simulink model "Sim_Multi"  (R2019b)
settings: Solver=VariableStepAuto  StartTime=0.0  StopTime=sim_time  FixedStep=t_sim  MaxStep=t_control  RelTol=1e-5  EnableMultiTasking=on
model workspace (MAT data in the model file):
  start_time = 1
values from neighbouring files (symbols this model uses):
  Att_init = [0;0;0] * d2r    [Init_Multi.m]
  Blade_flapping = 0    [Init_Multi.m]
  C_D = 0.40    (= 0.4)    [Init_Multi.m]
  CoG_nominal = [0;0;0.001]    [Init_Multi.m]
  CoG_real = [0;0;0.001]    [Init_Multi.m]
  Coriolis_correction = 0    [Init_Multi.m]
  d2r = pi/180    (= 0.0174532925199)    [Init_Multi.m]
  Dyn_thrust = 0    [Init_Multi.m]
  g = 9.80665    [Init_Multi.m]
  J_nominal = [Jxx Jxy Jxz;Jyx Jyy Jyz;Jzx Jzy Jzz]    [Init_Multi.m]
  J_real = [Jxx Jxy Jxz;Jyx Jyy Jyz;Jzx Jzy Jzz]    [Init_Multi.m]
  k1 = -1.125    [Init_Multi.m]
  k2 = -1.372    [Init_Multi.m]
  k3 = -1.718    [Init_Multi.m]
  k4 = -0.655    [Init_Multi.m]
  k_a1s = 1.5 / 4.0    (= 0.375)    [Init_Multi.m]
  k_beta = 0.23    [Init_Multi.m]
  kappa = 1.00    (= 1)    [Init_Multi.m]
  mass_nominal = 0.550    (= 0.55)    [Init_Multi.m]
  mass_real = 0.550    (= 0.55)    [Init_Multi.m]
  max_thrust = max_thrust + (MotorMatrix_nominal(i,7)*MotorMatrix_nominal(i,12)+MotorMatrix_nominal(i,8)*MotorMatrix_nominal(i,12)^2)    [Init_Multi.m]
  MaxRate_cmd = [360;360;120] * d2r    [Init_Multi.m]
  min_thrust = min_thrust + (MotorMatrix_nominal(i,7)*MotorMatrix_nominal(i,11)+MotorMatrix_nominal(i,8)*MotorMatrix_nominal(i,11)^2)    [Init_Multi.m]
  MotorMap = B' * inv(B * B')    [Init_Multi.m]
  MotorMatrix_nominal = [045 , 0.170 , -0.028 , -1 , 1.0 , 0.010 , [9.6820 , 0.010872]*1e-5 , [1.4504 , 0.0016312]*1e-6 , 0000 , 6000 , [0.0 , 0.0 , 0.0] , 8*2.54/100 , 11/1000;                         135 , 0.170 , -0.028 , +1 , 1.0 , 0.010 , [9.6820 , 0.010872]*1e-5 , [1.4504 , 0.0016312]*1e-6 , 0000 , 6000 , [0.0 , 0.0 , 0.0] , 8*2.54/100 , 11/1000;                         225 , 0.170 , -0.028 , -1 , 1.0 , 0.010 , [9. ...(+284 chars)    [Init_Multi.m]
  MotorMatrix_real = [045 , 0.170 , -0.028 , -1 , 1.0 , 0.010 , [9.6820 , 0.010872]*1e-5 , [1.4504 , 0.0016312]*1e-6 , 0000 , 6000 , [0.0 , 0.0 , 0.0] , 8*2.54/100 , 11/1000;                      135 , 0.170 , -0.028 , +1 , 1.0 , 0.010 , [9.6820 , 0.010872]*1e-5 , [1.4504 , 0.0016312]*1e-6 , 0000 , 6000 , [0.0 , 0.0 , 0.0] , 8*2.54/100 , 11/1000;                      225 , 0.170 , -0.028 , -1 , 1.0 , 0.010 , [9.6820 , ...(+275 chars)    [Init_Multi.m]
  Noise_flag = 1    [Init_Multi.m]
  omega_init = [0;0;0]    [Init_Multi.m]
  q_init = rpy2quat(Att_init)    [Init_Multi.m]
  r2d = 180/pi    (= 57.2957795131)    [Init_Multi.m]
  rho = 1.225    [Init_Multi.m]
  rpm2radpersec = 2*pi/60    (= 0.10471975512)    [Init_Multi.m]
  rpm_init = 3104.5025852    [Init_Multi.m]
  Surface_params = [a;b;c]    [Init_Multi.m]
  t_control = t_control_2*4    (= 0.02)    [Init_Multi.m]
  t_sim = 1/1000    (= 0.001)    [Init_Multi.m]
  thrust_reserve = 0.10    (= 0.1)    [Init_Multi.m]
  v_h = 4.0    (= 4)    [Init_Multi.m]
  Vb_init = [0;0;0]    [Init_Multi.m]
  Vi_init = R_IB_init' * Vb_init    [Init_Multi.m]
  Xi_init = [0;0;-1]    [Init_Multi.m]
undefined symbols (not defined in the file or in its folder): anti_windup_1, anti_windup_2, DiscIntNeverNeededParam, Kd_1, Kd_2, Kff_1, Kff_2, Ki_1, Ki_2, Kp_1, Kp_2, Kpass_1, magnitude, rpy2quat, thrust2rpm
libraries: simulink x35, dspsigops x3, sharedtransform x2, dspmtrx3 x1, robotuavlib x1, vrlib x1
(part 1 of 4)
settings Model: SimulationMode=accelerator  Creator=JV  LastModifiedBy=max_g
settings DataIOCC: LimitDataPoints=on  SaveFormat=Array  ReturnWorkspaceOutputs=off
settings OptimizationCC: ExpressionDepthLimit=2147483647  InitFltsAndDblsToZero=on  LifeSpan=inf
settings DebuggingCC: UnderspecifiedInitializationDetection=Classic  MergeDetectMultiDrivingBlocksExec=none  SolverPrmCheckMsg=warning  FcnCallInpInsideContextMsg=warning  StateNameClashWarn=warning  SFUnexpectedBacktrackingDiag=warning  SFNoUnconditionalDefaultTransitionDiag=warning  SFExecutionAtInitializationDiag=none  ArithmeticOperatorsInVariantConditions=warning
settings HardwareCC: ProdBitPerPointer=32  ProdBitPerSizeT=32  ProdBitPerPtrDiffT=32  ProdLargestAtomicFloat=None  ProdIntDivRoundTo=Undefined  ProdEndianess=Unspecified  ProdWordSize=32  ProdHWDeviceType=32-bit Generic
settings ModelReferenceCC: PropagateSignalLabelsOutOfModel=off
settings SFSimCC: SimUseLocalCustomCode=off  CustomCodeUndefinedFunction=UseInterfaceOnly
settings RTWCC: RTWUseLocalCustomCode=off
settings CodeAppCC: StateflowObjectComments=on
settings GRTTargetCC: TargetLangStandard=C89/C90 (ANSI)  GeneratePreprocessorConditionals=Disable all  CombineOutputUpdateFcns=off  GRTInterface=on
settings ConfigComp: CovMetricSettings=dw  CovHtmlReporting=on  CovSaveCumulativeToWorkspaceVar=on  CovSaveSingleToWorkspaceVar=on  CovExternalEMLEnable=off  CovSFcnEnable=off

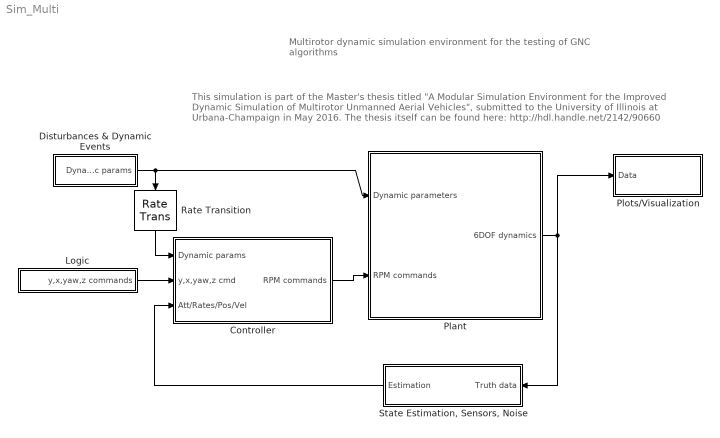
== system Sim_Multi ==
  note: This simulation is part of the Master's thesis titled "A Modular Simulation Environment for the Improved Dynamic Simulation
      | of Multirotor Unmanned Aerial Vehicles", submitted to the University of Illinois at Urbana-Champaign in May 2016.
      | The thesis itself can be found here: http://hdl.handle.net/2142/90660
  note: Multirotor dynamic simulation environment
      | for the testing of GNC algorithms
  Controller : Subsystem
  Disturbances & Dynamic Events : Subsystem
  Logic : Subsystem
  Plant : Subsystem
  Plots/Visualization : Subsystem
  Rate Transition : RateTransition  OutPortSampleTime=t_control_2
  "State Estimation, Sensors, Noise" : Subsystem
  wires:
  Plant/1(6DOF dynamics) -> "State Estimation, Sensors, Noise"/1(Truth data), Plots/Visualization/1(Data)
  Logic/1(y,x,yaw,z commands) -> Controller/2(y,x,yaw,z cmd)
  "State Estimation, Sensors, Noise"/1(Estimation) -> Controller/3(Att/Rates/Pos/Vel)
  Controller/1(RPM commands) -> Plant/2(RPM commands)
  Disturbances & Dynamic Events/1(Dynamic params) -> Plant/1(Dynamic parameters), Rate Transition/1
  Rate Transition/1 -> Controller/1(Dynamic params)

== system Sim_Multi/Controller ==
  note: All system parameters used in this block are the nominal parameters
      | that the controller is given about the system.
      | The true parameters of the dynamic system such as mass, inertia,
      | motor mapping matrix, ... may differ from these values.
  Dynamic params : Inport
  y,x,yaw,z cmd : Inport  Port=2
  Att/Rates/Pos/Vel : Inport  Port=3
  Controller Structure : Subsystem
  Mapping thrust to rpm and saturation : Subsystem
  Motor mapping : Subsystem
  Reshape : Reshape  OutputDimensionality=Column vector (2-D)
  RPM commands : Outport
  tag scope: RPM_commands=global
  wires:
  Att/Rates/Pos/Vel/1 -> Controller Structure/2(Att/Rates/Pos/Vel)
  Controller Structure/1(Torques/thrust cmd) -> Motor mapping/1(Torques/thrust cmd)
  y,x,yaw,z cmd/1 -> Controller Structure/1(y,x,yaw,z cmd)
  Reshape/1 -> RPM commands/1
  Dynamic params/1 -> Controller Structure/3(Dynamic params), Mapping thrust to rpm and saturation/2(Dynamic parameters)
  Mapping thrust to rpm and saturation/1(RPM_cmd) -> [RPM_commands], Reshape/1
  Motor mapping/1(Thrust cmds) -> Mapping thrust to rpm and saturation/1(Thrust_cmds)

== system Sim_Multi/Disturbances & Dynamic Events ==
  Bus Creator : BusCreator  Inputs=12
  Constant : Constant  Value=MotorMatrix_real
  Constant1 : Constant  Value=CoG_real
  Constant2 : Constant  Value=mass_real
  Constant3 : Constant  Value=J_real
  Constant4 : Constant  Value=MotorMatrix_nominal
  Constant5 : Constant  Value=CoG_nominal
  Constant6 : Constant  Value=mass_nominal
  Constant7 : Constant  Value=J_nominal
  Disturbance (forces) : Constant  Value=0*[1;1;1]
  Disturbance (torques) : Constant  Value=0*[1;1;1]
  Rate Transition : RateTransition  OutPortSampleTime=t_sim
  Surface area params : Constant  Value=Surface_params
  Wind vector : Constant  Value=[0;0;0]
  Dynamic params : Outport
  wires:
  Bus Creator/1 -> Rate Transition/1
  Constant/1 -> Bus Creator/1  "MotorMatrix_real"
  Constant1/1 -> Bus Creator/2  "CoG_real"
  Constant2/1 -> Bus Creator/3  "mass_real"
  Constant3/1 -> Bus Creator/4  "J_real"
  Surface area params/1 -> Bus Creator/12  "Surface_params"
  Disturbance (torques)/1 -> Bus Creator/11  "Moment_disturb"
  Disturbance (forces)/1 -> Bus Creator/10  "Force_disturb"
  Wind vector/1 -> Bus Creator/9  "Wind_i"
  Constant4/1 -> Bus Creator/5  "MotorMatrix_nominal"
  Constant5/1 -> Bus Creator/6  "CoG_nominal"
  Constant6/1 -> Bus Creator/7  "mass_nominal"
  Constant7/1 -> Bus Creator/8  "J_nominal"
  Rate Transition/1 -> Dynamic params/1

== system Sim_Multi/Logic ==
  Rate commands : Subsystem
  y,x,yaw,z commands : Outport
  wires:
  Rate commands/1(Commands) -> y,x,yaw,z commands/1

== system Sim_Multi/Plant ==
  Dynamic parameters : Inport
  RPM commands : Inport  Port=2
  6DOF model : Subsystem
  Bus Creator : BusCreator  Inputs=10
  Bus Selector : BusSelector  OutputSignals=mass_real,J_real
  Force/Moment computation : Subsystem
  Rate Transition : RateTransition  OutPortSampleTime=t_sim
  Rate Transition1 : RateTransition  InitialCondition=rpm_init  OutPortSampleTime=t_sim
  Rate Transition2 : RateTransition  OutPortSampleTime=t_sim
  6DOF dynamics : Outport
  wires:
  RPM commands/1 -> Rate Transition1/1
  Bus Creator/1 -> Rate Transition2/1
  Dynamic parameters/1 -> Rate Transition/1
  6DOF model/1(X_i [m]) -> Bus Creator/1  "X_i"
  6DOF model/2(V_i [m/s]) -> Bus Creator/2  "V_i"
  6DOF model/3(V_b [m/s]) -> Bus Creator/3  "V_b"
  6DOF model/4(a_b [m/s^2]) -> Bus Creator/4  "a_b"
  Bus Selector/2 -> 6DOF model/4(Inertia [kgm^2])  "<J_real>"
  Bus Selector/1 -> 6DOF model/3(Mass [kg])  "<mass_real>"
  Force/Moment computation/1(Total forces) -> 6DOF model/1(Forces [N])
  Force/Moment computation/2(Total moments) -> 6DOF model/2(Moments [Nm])
  Rate Transition1/1 -> Force/Moment computation/2(RPM commands)
  Rate Transition/1 -> Bus Selector/1, Force/Moment computation/3(Dynamic parameters)
  6DOF model/5(a_i [m/s^2]) -> Bus Creator/5  "a_i"
  6DOF model/6(DCM_ib) -> Bus Creator/6  "DCM_ib"
  6DOF model/7(Quaternion q) -> Bus Creator/7  "Quat q"
  6DOF model/8(Euler [rad]) -> Bus Creator/8  "Euler"
  6DOF model/9(omega [rad/s]) -> Bus Creator/9  "omega"
  6DOF model/10(omega_dot [rad/s^2]) -> Bus Creator/10  "omega_dot"
  Rate Transition2/1 -> Force/Moment computation/1(6DOF dynamics), 6DOF dynamics/1

== system Sim_Multi/Plots//Visualization ==
  note: roll pitch yaw
  Data : Inport
  EulerAnglesScope : Scope  NumInputPorts=3
  MotorRPM : Scope  NumInputPorts=2
  PosScope : Scope  NumInputPorts=3
  QuatScope : Scope  NumInputPorts=4
  Rate Transition2 : RateTransition  Commented=through
  RatesScope : Scope  NumInputPorts=3
  Subsystem : Subsystem
  Subsystem1 : Subsystem
  Subsystem2 : Subsystem
  Subsystem3 : Subsystem
  Subsystem5 : Subsystem
  UAV Animation : robotuavlib/UAV Animation  UAVType=Multirotor  UAVSize=1  InertialZDirection=Down  SampleTime=-1  mask(robotics.sluav.internal.system.UAVAnimation){}
      settings: SourceProductName=Robotics System Toolbox UAV Library  SourceProductBaseCode=ROBOTICS_UAV_LIB
  VR Sink : vrlib/VR Sink  Commented=on  InstantiateOnLoad=on  SampleTime=0.1  ViewEnable=on  RemoteChange=off  RemoteView=on  AutoView=off  VideoDimensions=[]  AllowVariableSize=off
      settings: SourceProductName=Simulink
  VelScope : Scope  NumInputPorts=3
  wires:
  Data/1 -> Subsystem3/1(In1), Subsystem1/1(In1), Subsystem5/1(In1), Subsystem2/1(In1), Subsystem/1(In1)
  Subsystem/1(phi) -> EulerAnglesScope/1
  Subsystem/2(theta) -> EulerAnglesScope/2
  Subsystem/3(psi) -> EulerAnglesScope/3
  Subsystem2/1(q0) -> QuatScope/1
  Subsystem2/2(q1) -> QuatScope/2
  Subsystem2/3(q2) -> QuatScope/3
  Subsystem2/4(q3) -> QuatScope/4
  Subsystem1/1(Vx) -> VelScope/1
  Subsystem1/2(Vy) -> VelScope/2
  Subsystem1/3(Vz) -> VelScope/3
  Subsystem3/2(Yi) -> PosScope/2
  Subsystem3/3(Zi) -> PosScope/3
  Subsystem3/1(Xi) -> PosScope/1
  Subsystem5/1(p) -> RatesScope/1
  Subsystem5/2(q) -> RatesScope/2
  Subsystem5/3(r) -> RatesScope/3
  [cmd] -> Subsystem5/2(In2)
  [RPM_commands] -> MotorRPM/2
  [RPM_motor] -> Rate Transition2/1
  Rate Transition2/1 -> MotorRPM/1
  Subsystem2/5(Output) -> UAV Animation/2
  Subsystem3/4(Output) -> UAV Animation/1

== system Sim_Multi/State Estimation, Sensors, Noise ==
  Truth data : Inport
  Rate Transition : RateTransition  OutPortSampleTime=t_control_2
  Sensor models : Subsystem
  State estimation : Subsystem
  Estimation : Outport
  wires:
  Sensor models/1(Corrupted) -> State estimation/1(Sensors)
  Truth data/1 -> Sensor models/1(Truth)
  State estimation/1(Att/Pos/Vel/Accel) -> Rate Transition/1
  Rate Transition/1 -> Estimation/1

== system Sim_Multi/Controller/Controller Structure ==
  y,x,yaw,z cmd : Inport
  Att/Rates/Pos/Vel : Inport  Port=2
  Dynamic params : Inport  Port=3
  Bus Selector : BusSelector  OutputSignals=J_nominal
  Pos/Vel Control : Subsystem
  Torques/thrust cmd : Outport
  tag scope: J_control=global
  wires:
  Dynamic params/1 -> Bus Selector/1
  Bus Selector/1 -> [J_control]  "<J_nominal>"
  Att/Rates/Pos/Vel/1 -> Pos/Vel Control/1(Att/Rates/Pos/Vel)
  y,x,yaw,z cmd/1 -> Pos/Vel Control/2(Pos/Vel Commands)
  Pos/Vel Control/1(Torques/Thrust) -> Torques/thrust cmd/1

== system Sim_Multi/Controller/Mapping thrust to rpm and saturation ==
  Thrust_cmds : Inport
  Dynamic parameters : Inport  Port=2
  Bus Selector1 : BusSelector  OutputSignals=MotorMatrix_nominal
  For Each Subsystem : Subsystem  TreatAsAtomicUnit=on
  RPM_cmd : Outport
  wires:
  Dynamic parameters/1 -> Bus Selector1/1
  Bus Selector1/1 -> For Each Subsystem/2(MotorMatrix_nominal)  "<MotorMatrix_nominal>"
  For Each Subsystem/1(RPM_cmd_sat) -> RPM_cmd/1
  Thrust_cmds/1 -> For Each Subsystem/1(Thrust_cmds)

== system Sim_Multi/Controller/Motor mapping ==
  note: Overall thrust command is limited to a range
      | of 10...90% of max thrust to still allow room
      | for torque demands needed for maneuvering
  note: The motor mapping matrix used here to transform body axis torque commands
      | into thrust commands for each motor is populated with the nominal arm length
      | and motor position information that the controller thinks are correct, not the
      | actual values used in the true dynamics computation block.
  Torques/thrust cmd : Inport
  Constant1 : Constant  Value=MotorMap
  Demux : Demux  Outputs=[3 1]
  Matrix Multiply1 : Product  Multiplication=Matrix(*)
  Max thrust limit : Subsystem
  Min thrust limit : Subsystem
  Mux : Mux  Inputs=2
  Rate Transition : RateTransition  Commented=through  OutPortSampleTime=t_control_2
  Saturation Dynamic : simulink/Discontinuities/Saturation Dynamic  OutMin=[]  OutMax=[]  OutDataTypeStr=Inherit: Same as second input  OutDataType=fixdt(1, 16)  OutScaling=2^-10  DoSatur=off
  Thrust cmds : Outport
  wires:
  Constant1/1 -> Matrix Multiply1/1
  Rate Transition/1 -> Thrust cmds/1  "These are thrust demands to each motor"
  Matrix Multiply1/1 -> Rate Transition/1
  Torques/thrust cmd/1 -> Demux/1
  Demux/2 -> Saturation Dynamic/2
  Min thrust limit/1(Out1) -> Saturation Dynamic/3
  Max thrust limit/1(Out1) -> Saturation Dynamic/1
  Saturation Dynamic/1 -> Mux/2
  Demux/1 -> Mux/1
  Mux/1 -> Matrix Multiply1/2

== system Sim_Multi/Logic/Rate commands ==
  note: planned waypoints plus jerk-minimizing trajectory generator
  Basic Jerk-minimized Trajectory Generator : Subsystem
  Mux : Mux
  Rate Transition : RateTransition  Integrity=off  OutPortSampleTime=t_control_2
  Scope2 : Scope  NumInputPorts=4
  Commands : Outport
  wires:
  Rate Transition/1 -> Commands/1
  Mux/1 -> Rate Transition/1
  Basic Jerk-minimized Trajectory Generator/1(Y) -> Mux/1, Scope2/1
  Basic Jerk-minimized Trajectory Generator/4(Z) -> Mux/4, Scope2/4
  Basic Jerk-minimized Trajectory Generator/2(X) -> Mux/2, Scope2/2
  Basic Jerk-minimized Trajectory Generator/3(yaw) -> Mux/3, Scope2/3

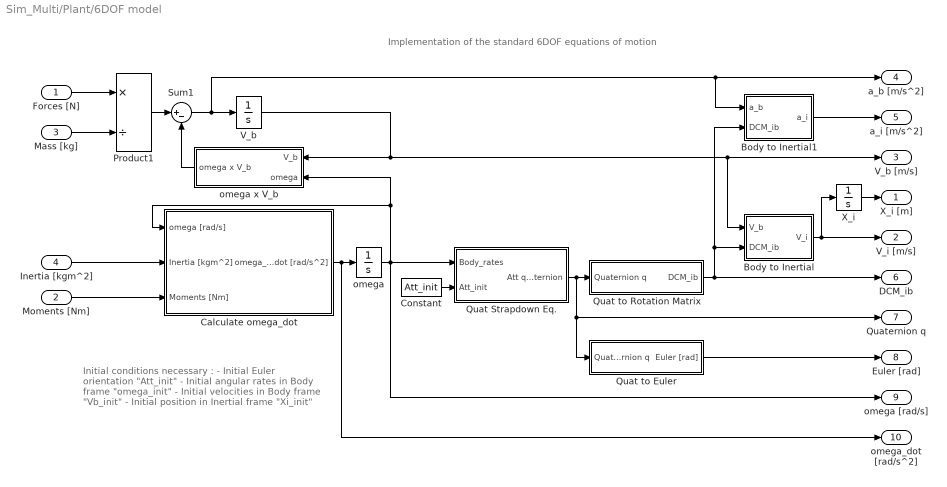
== system Sim_Multi/Plant/6DOF model ==
  note: Implementation of the standard 6DOF equations of motion
  note: Initial conditions necessary :
      | - Initial Euler orientation "Att_init"
      | - Initial angular rates in Body frame "omega_init"
      | - Initial velocities in Body frame "Vb_init"
      | - Initial position in Inertial frame "Xi_init"
  Forces [N] : Inport
  Moments [Nm] : Inport  Port=2
  Mass [kg] : Inport  Port=3
  Inertia [kgm^2] : Inport  Port=4
  Body to Inertial : Subsystem
  Body to Inertial1 : Subsystem
  Calculate omega_dot : Subsystem
  Constant : Constant  Value=Att_init
  Product1 : Product  Inputs=*/  SaturateOnIntegerOverflow=on  OutDataTypeStr=Inherit: Same as first input
  Quat Strapdown Eq. : Subsystem
  Quat to Euler : Subsystem
  Quat to Rotation Matrix : Subsystem
  Sum1 : Sum  Inputs=|+-  SaturateOnIntegerOverflow=on
  V_b : Integrator  InitialCondition=Vb_init
  X_i : Integrator  InitialCondition=Xi_init
  omega : Integrator  InitialCondition=omega_init
  omega x V_b : Subsystem
  X_i [m] : Outport
  V_i [m/s] : Outport  Port=2
  V_b [m/s] : Outport  Port=3
  a_b [m/s^2] : Outport  Port=4
  a_i [m/s^2] : Outport  Port=5
  DCM_ib : Outport  Port=6
  Quaternion q : Outport  Port=7
  Euler [rad] : Outport  Port=8
  omega [rad/s] : Outport  Port=9
  omega_dot [rad/s^2] : Outport  Port=10
  wires:
  Forces [N]/1 -> Product1/1
  Mass [kg]/1 -> Product1/2
  Product1/1 -> Sum1/1
  omega x V_b/1(omega x V_b) -> Sum1/2
  V_b/1 -> V_b [m/s]/1, Body to Inertial/1(V_b), omega x V_b/1(V_b)
  Inertia [kgm^2]/1 -> Calculate omega_dot/2(Inertia [kgm^2])
  Moments [Nm]/1 -> Calculate omega_dot/3(Moments [Nm])
  Calculate omega_dot/1(omega_dot [rad/s^2]) -> omega_dot [rad/s^2]/1, omega/1
  omega/1 -> Calculate omega_dot/1(omega [rad/s]), omega x V_b/2(omega), omega [rad/s]/1, Quat Strapdown Eq./1(Body_rates)
  Quat Strapdown Eq./1(Att quaternion) -> Quat to Euler/1(Quaternion q), Quaternion q/1, Quat to Rotation Matrix/1(Quaternion q)
  Quat to Euler/1(Euler [rad]) -> Euler [rad]/1
  Body to Inertial/1(V_i) -> V_i [m/s]/1, X_i/1
  X_i/1 -> X_i [m]/1
  Constant/1 -> Quat Strapdown Eq./2(Att_init)
  Quat to Rotation Matrix/1(DCM_ib) -> Body to Inertial1/2(DCM_ib), Body to Inertial/2(DCM_ib), DCM_ib/1
  Body to Inertial1/1(a_i) -> a_i [m/s^2]/1
  Sum1/1 -> V_b/1, a_b [m/s^2]/1, Body to Inertial1/1(a_b)

== system Sim_Multi/Plant/Force//Moment computation ==
  note: Computation of all forces and moments acting on the airframe
  6DOF dynamics : Inport
  RPM commands : Inport  Port=2
  Dynamic parameters : Inport  Port=3
  Bus Selector : BusSelector  OutputSignals=Force_disturb,Moment_disturb
  Compute aerodynamic drag of the airframe in Body axes : Subsystem
  Compute force of gravity in Body axes : Subsystem
  Forces and moments generated by spinning propellers : Subsystem
  Ground contact forces and moments in Body axes : Subsystem
  Rate Transition : RateTransition  OutPortSampleTime=t_sim
  Sum{,1..3} (4 alike) : Sum  Inputs=|++
  Terminator : Terminator
  Terminator1 : Terminator
  Total forces : Outport
  Total moments : Outport  Port=2
  wires:
  RPM commands/1 -> Forces and moments generated by spinning propellers/1(RPM_commands)
  6DOF dynamics/1 -> Rate Transition/1
  Forces and moments generated by spinning propellers/2(Motor forces) -> Sum/1
  Compute force of gravity in Body axes/1(Gravity force) -> Sum/2
  Dynamic parameters/1 -> Ground contact forces and moments in Body axes/2(Dynamic parameters), Bus Selector/1, Compute aerodynamic drag of the airframe in Body axes/2(Dynamic parameters), Compute force of gravity in Body axes/2(Dynamic parameters), Forces and moments generated by spinning propellers/2(Dynamic parameters)
  Bus Selector/1 -> Sum1/2  "<Force_disturb>"
  Bus Selector/2 -> Sum2/2  "<Moment_disturb>"
  Forces and moments generated by spinning propellers/1(Motor moments) -> Sum2/1
  Sum/1 -> Sum3/1
  Sum3/1 -> Sum1/1
  Compute aerodynamic drag of the airframe in Body axes/1(Drag force) -> Sum3/2
  Rate Transition/1 -> Forces and moments generated by spinning propellers/3(6DOF dynamics), Compute aerodynamic drag of the airframe in Body axes/1(6DOF dynamics), Ground contact forces and moments in Body axes/1(6DOF dynamics), Compute force of gravity in Body axes/1(6DOF dynamics)
  Sum1/1 -> Total forces/1
  Sum2/1 -> Total moments/1
  Ground contact forces and moments in Body axes/1(Ground moments) -> Terminator/1
  Ground contact forces and moments in Body axes/2(Ground forces) -> Terminator1/1

== system Sim_Multi/Plots//Visualization/Subsystem ==
  In1 : Inport
  Bus Selector : BusSelector  OutputSignals=Euler
  Demux : Demux  Outputs=3
  Gain : Gain  Gain=r2d
  phi : Outport
  theta : Outport  Port=2
  psi : Outport  Port=3
  wires:
  Bus Selector/1 -> Gain/1  "<Euler>"
  In1/1 -> Bus Selector/1
  Gain/1 -> Demux/1
  Demux/1 -> phi/1
  Demux/2 -> theta/1
  Demux/3 -> psi/1

== system Sim_Multi/Plots//Visualization/Subsystem1 ==
  In1 : Inport
  Bus Selector : BusSelector  OutputSignals=V_i
  Demux4 : Demux  Outputs=3
  Vx : Outport
  Vy : Outport  Port=2
  Vz : Outport  Port=3
  wires:
  Bus Selector/1 -> Demux4/1  "<V_i>"
  In1/1 -> Bus Selector/1
  Demux4/1 -> Vx/1
  Demux4/2 -> Vy/1
  Demux4/3 -> Vz/1

== system Sim_Multi/Plots//Visualization/Subsystem2 ==
  In1 : Inport
  Bus Selector : BusSelector  OutputSignals=Quat q
  Demux5 : Demux
  Mux : Mux
  q0 : Outport
  q1 : Outport  Port=2
  q2 : Outport  Port=3
  q3 : Outport  Port=4
  Output : Outport  Port=5
  wires:
  Bus Selector/1 -> Demux5/1  "<Quat q>"
  In1/1 -> Bus Selector/1
  Demux5/1 -> Mux/1, q0/1
  Demux5/2 -> q1/1, Mux/2
  Demux5/3 -> Mux/3, q2/1
  Demux5/4 -> Mux/4, q3/1
  Mux/1 -> Output/1

== system Sim_Multi/Plots//Visualization/Subsystem3 ==
  In1 : Inport
  Bus Selector : BusSelector  OutputSignals=X_i
  Demux4 : Demux  Outputs=3
  Mux : Mux  Inputs=3
  Xi : Outport
  Yi : Outport  Port=2
  Zi : Outport  Port=3
  Output : Outport  Port=4
  wires:
  Bus Selector/1 -> Demux4/1  "<X_i>"
  In1/1 -> Bus Selector/1
  Demux4/1 -> Mux/1, Xi/1
  Demux4/2 -> Mux/2, Yi/1
  Demux4/3 -> Mux/3, Zi/1
  Mux/1 -> Output/1

== system Sim_Multi/Plots//Visualization/Subsystem5 ==
  In1 : Inport
  In2 : Inport  Port=2
  Bus Selector : BusSelector  OutputSignals=omega
  Demux : Demux  Outputs=3
  Demux1 : Demux  Outputs=3
  Mux : Mux  Inputs=2
  Mux1 : Mux  Inputs=2
  Mux2 : Mux  Inputs=2
  Rate Transition : RateTransition  OutPortSampleTime=t_sim
  p : Outport
  q : Outport  Port=2
  r : Outport  Port=3
  wires:
  Bus Selector/1 -> Demux/1  "<omega>"
  Demux/1 -> Mux1/1
  Demux1/1 -> Mux1/2
  Demux/2 -> Mux/1
  Demux1/2 -> Mux/2
  Demux/3 -> Mux2/1
  Demux1/3 -> Mux2/2
  In1/1 -> Bus Selector/1
  In2/1 -> Rate Transition/1
  Mux1/1 -> p/1
  Mux/1 -> q/1
  Mux2/1 -> r/1
  Rate Transition/1 -> Demux1/1

== system Sim_Multi/State Estimation, Sensors, Noise/Sensor models ==
  note: The available sensor outputs are body rates and body accelerations.
      | In the simple case, noise is added to the rate and accel outputs of the 6DOF block to 'simulate' sensor output.
  Truth : Inport
  Acc noise : Subsystem
  Bus Creator : BusCreator  Inputs=9
  Bus Selector : BusSelector  OutputSignals=a_b,omega
  Bus Selector1 : BusSelector  OutputSignals=X_i,V_i,V_b,DCM_ib,Quat q,Euler,omega_dot
  Gain : Gain
  Gain1 : Gain
  Gyro noise : Subsystem
  Noisy acc : Scope
  Noisy omega : Scope
  Sum : Sum
  Sum1 : Sum
  Corrupted : Outport
  wires:
  Truth/1 -> Bus Selector/1, Bus Selector1/1
  Bus Creator/1 -> Corrupted/1
  Sum/1 -> Noisy omega/1, Gain/1  "omega"
  Sum1/1 -> Noisy acc/1, Gain1/1  "a_b"
  Bus Selector1/1 -> Bus Creator/1  "<X_i>"
  Bus Selector1/2 -> Bus Creator/2  "<V_i>"
  Bus Selector1/3 -> Bus Creator/3  "<V_b>"
  Acc noise/1(Noise) -> Sum1/1
  Bus Selector/1 -> Sum1/2  "<a_b>"
  Gain1/1 -> Bus Creator/4  "a_b"
  Bus Selector1/4 -> Bus Creator/5  "<DCM_ib>"
  Bus Selector1/5 -> Bus Creator/6  "<Quat q>"
  Bus Selector1/6 -> Bus Creator/7  "<Euler>"
  Gyro noise/1(Noise) -> Sum/2
  Bus Selector/2 -> Sum/1  "<omega>"
  Gain/1 -> Bus Creator/8  "omega"
  Bus Selector1/7 -> Bus Creator/9  "<omega_dot>"

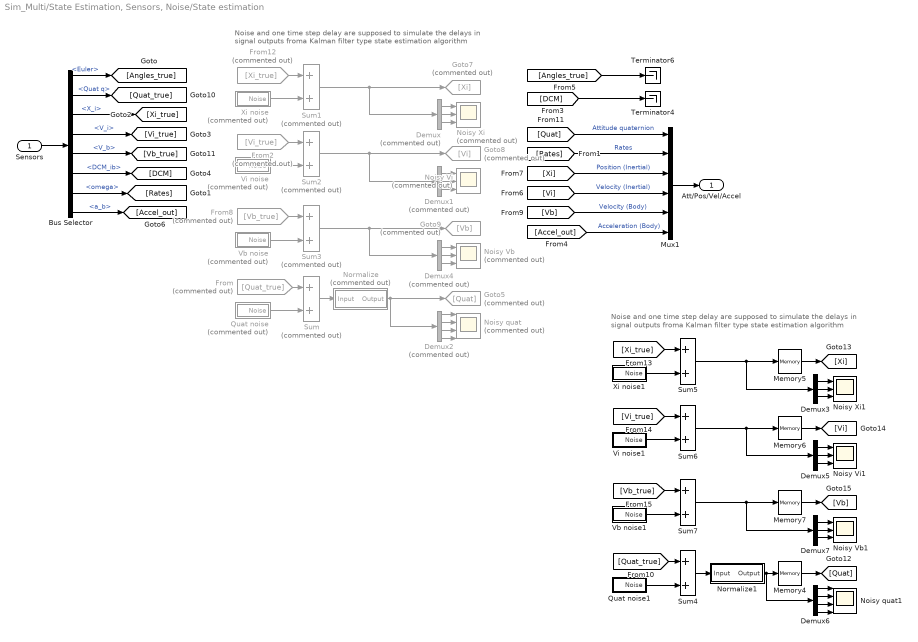
== system Sim_Multi/State Estimation, Sensors, Noise/State estimation ==
  note: Noise and one time step delay are supposed to simulate the delays
      | in signal outputs froma Kalman filter type state estimation algorithm
  note: Noise and one time step delay are supposed to simulate the delays
      | in signal outputs froma Kalman filter type state estimation algorithm
  Sensors : Inport
  Bus Selector : BusSelector  OutputSignals=Euler,Quat q,X_i,V_i,V_b,DCM_ib,omega,a_b
  Demux : Demux  Commented=on  Outputs=3
  Demux1 : Demux  Commented=on  Outputs=3
  Demux2 : Demux  Commented=on
  Demux3 : Demux  Outputs=3
  Demux4 : Demux  Commented=on  Outputs=3
  Demux5 : Demux  Outputs=3
  Demux6 : Demux
  Demux7 : Demux  Outputs=3
  From : From  Commented=on  GotoTag=Quat_true
  From12 : From  Commented=on  GotoTag=Xi_true
      settings: CloseFcn=tagdialog Close
  From2 : From  Commented=on  GotoTag=Vi_true
      settings: CloseFcn=tagdialog Close
  From8 : From  Commented=on  GotoTag=Vb_true
      settings: CloseFcn=tagdialog Close
  Goto5 : Goto  Commented=on  GotoTag=Quat
  Goto7 : Goto  Commented=on  GotoTag=Xi
  Goto8 : Goto  Commented=on  GotoTag=Vi
  Goto9 : Goto  Commented=on  GotoTag=Vb
  Memory4 : Memory  InitialCondition=q_init  InheritSampleTime=on  LinearizeAsDelay=on
  Memory5 : Memory  InitialCondition=Xi_init  InheritSampleTime=on  LinearizeAsDelay=on
  Memory6 : Memory  InitialCondition=Vi_init  InheritSampleTime=on  LinearizeAsDelay=on
  Memory7 : Memory  InitialCondition=Vi_init  InheritSampleTime=on  LinearizeAsDelay=on
  Mux1 : Mux  Inputs=6
  Noisy Vb : Scope  Commented=on  NumInputPorts=3
  Noisy Vb1 : Scope  NumInputPorts=3
  Noisy Vi : Scope  Commented=on  NumInputPorts=3
  Noisy Vi1 : Scope  NumInputPorts=3
  Noisy Xi : Scope  Commented=on  NumInputPorts=3
  Noisy Xi1 : Scope  NumInputPorts=3
  Noisy quat : Scope  Commented=on  NumInputPorts=4
  Noisy quat1 : Scope  NumInputPorts=4
  Normalize : Subsystem  Commented=on
  Normalize1 : Subsystem
  Quat noise : Subsystem  Commented=on
  Quat noise1 : Subsystem
  Sum{,1..3} (4 alike) : Sum  Commented=on
  Sum{4..7} (4 alike) : Sum
  Terminator4 : Terminator
  Terminator6 : Terminator
  Vb noise : Subsystem  Commented=on
  Vb noise1 : Subsystem
  Vi noise : Subsystem  Commented=on
  Vi noise1 : Subsystem
  Xi noise : Subsystem  Commented=on
  Xi noise1 : Subsystem
  Att/Pos/Vel/Accel : Outport
  wires:
  Sensors/1 -> Bus Selector/1
  Bus Selector/3 -> [Xi_true]  "<X_i>"
  Bus Selector/4 -> [Vi_true]  "<V_i>"
  Bus Selector/6 -> [DCM]  "<DCM_ib>"
  Bus Selector/7 -> [Rates]  "<omega>"
  Bus Selector/8 -> [Accel_out]  "<a_b>"
  Bus Selector/1 -> [Angles_true]  "<Euler>"
  [Quat] -> Mux1/1  "Attitude quaternion"
  [Rates] -> Mux1/2  "Rates"
  Bus Selector/2 -> [Quat_true]  "<Quat q>"
  [DCM] -> Terminator4/1
  [Angles_true] -> Terminator6/1
  Sum/1 -> Normalize/1(Input)
  Quat noise/1(Noise) -> Sum/2
  From/1 -> Sum/1
  Normalize/1(Output) -> Goto5/1, Demux2/1
  Xi noise/1(Noise) -> Sum1/2
  Sum1/1 -> Goto7/1, Demux/1
  From12/1 -> Sum1/1
  Vi noise/1(Noise) -> Sum2/2
  Sum2/1 -> Goto8/1, Demux1/1
  From2/1 -> Sum2/1
  [Xi] -> Mux1/3  "Position (Inertial)"
  [Vi] -> Mux1/4  "Velocity (Inertial)"
  Mux1/1 -> Att/Pos/Vel/Accel/1
  Demux/1 -> Noisy Xi/1
  Demux/2 -> Noisy Xi/2
  Demux/3 -> Noisy Xi/3
  Demux1/1 -> Noisy Vi/1
  Demux1/2 -> Noisy Vi/2
  Demux1/3 -> Noisy Vi/3
  Demux2/1 -> Noisy quat/1
  Demux2/2 -> Noisy quat/2
  Demux2/3 -> Noisy quat/3
  Demux2/4 -> Noisy quat/4
  Vb noise/1(Noise) -> Sum3/2
  Sum3/1 -> Goto9/1, Demux4/1
  From8/1 -> Sum3/1
  Demux4/1 -> Noisy Vb/1
  Demux4/2 -> Noisy Vb/2
  Demux4/3 -> Noisy Vb/3
  Bus Selector/5 -> [Vb_true]  "<V_b>"
  [Vb] -> Mux1/5  "Velocity (Body)"
  [Accel_out] -> Mux1/6  "Acceleration (Body)"
  Sum7/1 -> Demux7/1, Memory7/1
  Demux7/3 -> Noisy Vb1/3
  Demux5/1 -> Noisy Vi1/1
  Demux3/2 -> Noisy Xi1/2
  Demux3/1 -> Noisy Xi1/1
  Vi noise1/1(Noise) -> Sum6/2
  Demux3/3 -> Noisy Xi1/3
  [Vi_true] -> Sum6/1
  [Xi_true] -> Sum5/1
  Memory4/1 -> [Quat]
  [Quat_true] -> Sum4/1
  Quat noise1/1(Noise) -> Sum4/2
  Demux7/2 -> Noisy Vb1/2
  [Vb_true] -> Sum7/1
  Memory6/1 -> [Vi]
  Sum4/1 -> Normalize1/1(Input)
  Normalize1/1(Output) -> Demux6/1, Memory4/1
  Demux6/1 -> Noisy quat1/1
  Demux6/2 -> Noisy quat1/2
  Demux7/1 -> Noisy Vb1/1
  Demux6/4 -> Noisy quat1/4
  Xi noise1/1(Noise) -> Sum5/2
  Memory5/1 -> [Xi]
  Demux5/2 -> Noisy Vi1/2
  Vb noise1/1(Noise) -> Sum7/2
  Demux5/3 -> Noisy Vi1/3
  Sum6/1 -> Demux5/1, Memory6/1
  Sum5/1 -> Demux3/1, Memory5/1
  Memory7/1 -> [Vb]
  Demux6/3 -> Noisy quat1/3

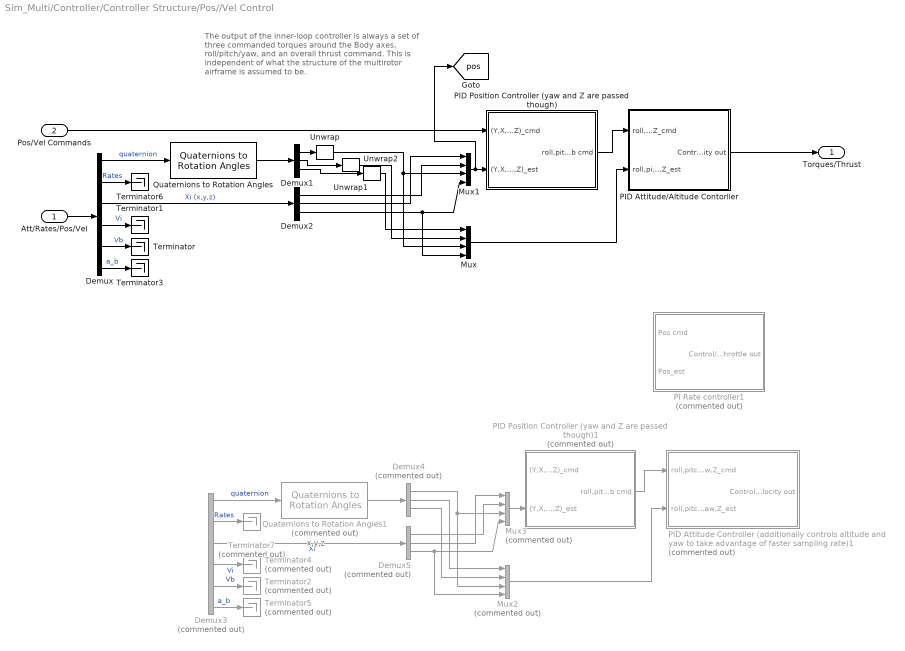
== system Sim_Multi/Controller/Controller Structure/Pos//Vel Control ==
  note: The output of the inner-loop controller is always
      | a set of three commanded torques around the
      | Body axes, roll/pitch/yaw, and an overall thrust
      | command.
      | This is independent of what the structure of the
      | multirotor airframe is assumed to be.
  note: x,y,z
  Att/Rates/Pos/Vel : Inport
  Pos/Vel Commands : Inport  Port=2
  Demux : Demux  Outputs=[4 3 3 3 3 3]
  Demux1 : Demux  Outputs=3
  Demux2 : Demux  Outputs=3
  Demux3 : Demux  Commented=on  Outputs=[4 3 3 3 3 3]
  Demux4 : Demux  Commented=on  Outputs=3
  Demux5 : Demux  Commented=on  Outputs=3
  Mux : Mux
  Mux1 : Mux
  Mux2 : Mux  Commented=on
  Mux3 : Mux  Commented=on
  PI Rate controller1 : Subsystem  Commented=on
  PID Attitude Controller (additionally controls altitude and yaw to take advantage of faster sampling rate)1 : Subsystem  Commented=on
  PID Attitude/Altitude Contorller : Subsystem
  PID Position Controller (yaw and Z are passed though) : Subsystem
  PID Position Controller (yaw and Z are passed though)1 : Subsystem  Commented=on
  Quaternions to Rotation Angles : sharedtransform/Quaternions to Rotation Angles  rotationOrder=ZYX  aMode=aMode
      settings: SourceProductBaseCode=AE
  Quaternions to Rotation Angles1 : sharedtransform/Quaternions to Rotation Angles  Commented=on  rotationOrder=ZYX  aMode=aMode
      settings: SourceProductBaseCode=AE
  Terminator{,1,3,6} (4 alike) : Terminator
  Terminator{2,4..5,7} (4 alike) : Terminator  Commented=on
  Unwrap : dspsigops/Unwrap  tol=pi/2  running=off
  Unwrap1 : dspsigops/Unwrap  tol=pi/2  running=off
  Unwrap2 : dspsigops/Unwrap  tol=pi/2  running=off
  Torques/Thrust : Outport
  tag scope: pos=global
  wires:
  Att/Rates/Pos/Vel/1 -> Demux/1
  Demux/4 -> Terminator1/1  "Vi"
  Demux/6 -> Terminator3/1  "a_b"
  Pos/Vel Commands/1 -> PID Position Controller (yaw and Z are passed though)/1((Y,X,yaw,Z)_cmd)
  Demux/2 -> Terminator6/1  "Rates"
  Demux/1 -> Quaternions to Rotation Angles/1  "quaternion"
  Quaternions to Rotation Angles/1 -> Demux1/1
  Mux1/1 -> [pos], PID Position Controller (yaw and Z are passed though)/2((Y,X,yaw,Z)_est)
  Demux/3 -> Demux2/1  "Xi (x,y,z)"
  Demux1/1 -> Unwrap/1
  Demux2/3 -> Mux/4, Mux1/4
  Demux2/2 -> Mux1/1
  Demux2/1 -> Mux1/2
  PID Position Controller (yaw and Z are passed though)/1(roll,pitch,yaw,climb cmd) -> PID Attitude/Altitude Contorller/1(roll,pitch,yaw,Z_cmd)
  PID Attitude/Altitude Contorller/1(Control/Velocity out) -> Torques/Thrust/1
  Mux/1 -> PID Attitude/Altitude Contorller/2(roll,pitch,yaw,Z_est)
  Demux/5 -> Terminator/1  "Vb"
  PID Position Controller (yaw and Z are passed though)1/1(roll,pitch,yaw,climb cmd) -> PID Attitude Controller (additionally controls altitude and yaw to take advantage of faster sampling rate)1/1(roll,pitch,yaw,Z_cmd)
  Demux3/2 -> Terminator7/1  "Rates"
  Demux4/2 -> Mux2/1
  Mux2/1 -> PID Attitude Controller (additionally controls altitude and yaw to take advantage of faster sampling rate)1/2(roll,pitch,yaw,Z_est)
  Demux4/3 -> Mux2/2
  Demux3/3 -> Demux5/1  "Xi"
  Mux3/1 -> PID Position Controller (yaw and Z are passed though)1/2((Y,X,yaw,Z)_est)
  Demux5/2 -> Mux3/1
  Demux5/3 -> Mux2/4, Mux3/4
  Demux3/6 -> Terminator5/1  "a_b"
  Demux5/1 -> Mux3/2
  Demux3/4 -> Terminator4/1  "Vi"
  Quaternions to Rotation Angles1/1 -> Demux4/1
  Demux4/1 -> Mux2/3, Mux3/3
  Demux3/5 -> Terminator2/1  "Vb"
  Demux3/1 -> Quaternions to Rotation Angles1/1  "quaternion"
  Unwrap/1 -> Mux1/3, Mux/3
  Demux1/2 -> Unwrap1/1
  Unwrap1/1 -> Mux/2
  Demux1/3 -> Unwrap2/1
  Unwrap2/1 -> Mux/1

== system Sim_Multi/Controller/Mapping thrust to rpm and saturation/For Each Subsystem ==
  note: The thrust commands from the controller are turned into RPM commands by solving the
      | nominal (quadratic) rpm to thrust equations for RPM.
      | These min and max RPM values are then saturated using the nominal min and max RPM
      | values given for the particular motor/propeller combination.
  Thrust_cmds : Inport  Partition=on  PartitionDimension=1  PartitionWidth=1  PartitionOffset=0
  MotorMatrix_nominal : Inport  Port=2  Partition=on  PartitionDimension=1  PartitionWidth=1  PartitionOffset=0
  For Each : ForEach  DisableCoverage=on
  Mux : Mux  Inputs=2
  Saturation Dynamic : simulink/Discontinuities/Saturation Dynamic  OutMin=[]  OutMax=[]  OutDataTypeStr=Inherit: Same as second input  OutDataType=fixdt(1, 16)  OutScaling=2^-10  DoSatur=off
  Saturation limit: no negative thrust : Saturate  UpperLimit=inf  LowerLimit=0
  Selector1 : Selector  InputPortWidth=17  IndexOptions=Index vector (dialog)  Indices=[11]  OutputSizes=1
  Selector2 : Selector  InputPortWidth=17  IndexOptions=Index vector (dialog)  Indices=[12]  OutputSizes=1
  Selector3 : Selector  InputPortWidth=17  IndexOptions=Index vector (dialog)  Indices=[7 8]  OutputSizes=1
  thrust2rpm : MATLABFcn  MATLABFcn=thrust2rpm(u)  OutputDimensions=1
  RPM_cmd_sat : Outport  ConcatenationDimension=1
  wires:
  Selector3/1 -> Mux/1  "Thrust params a1 and a2"
  Thrust_cmds/1 -> Saturation limit: no negative thrust/1
  Mux/1 -> thrust2rpm/1
  thrust2rpm/1 -> Saturation Dynamic/2  "Commanded RPM value for each motor"
  Selector2/1 -> Saturation Dynamic/1  "Nominal max RPM"
  Selector1/1 -> Saturation Dynamic/3  "Nominal min RPM"
  Saturation Dynamic/1 -> RPM_cmd_sat/1
  MotorMatrix_nominal/1 -> Selector1/1, Selector2/1, Selector3/1
  Saturation limit: no negative thrust/1 -> Mux/2

== system Sim_Multi/Controller/Motor mapping/Max thrust limit ==
  Constant : Constant  Value=max_thrust
  Constant2 : Constant  Value=min_thrust
  Gain : Gain  Gain=thrust_reserve
  Sum : Sum  Inputs=|+-
  Sum1 : Sum  Inputs=+-|
  Out1 : Outport
  wires:
  Constant/1 -> Sum1/1, Sum/1
  Sum1/1 -> Out1/1
  Constant2/1 -> Sum/2
  Sum/1 -> Gain/1
  Gain/1 -> Sum1/2

== system Sim_Multi/Controller/Motor mapping/Min thrust limit ==
  Constant : Constant  Value=max_thrust
  Constant2 : Constant  Value=min_thrust
  Gain : Gain  Gain=thrust_reserve
  Sum : Sum  Inputs=|+-
  Sum1 : Sum  Inputs=|++
  Out1 : Outport
  wires:
  Constant/1 -> Sum/1
  Sum1/1 -> Out1/1
  Constant2/1 -> Sum1/2, Sum/2
  Sum/1 -> Gain/1
  Gain/1 -> Sum1/1

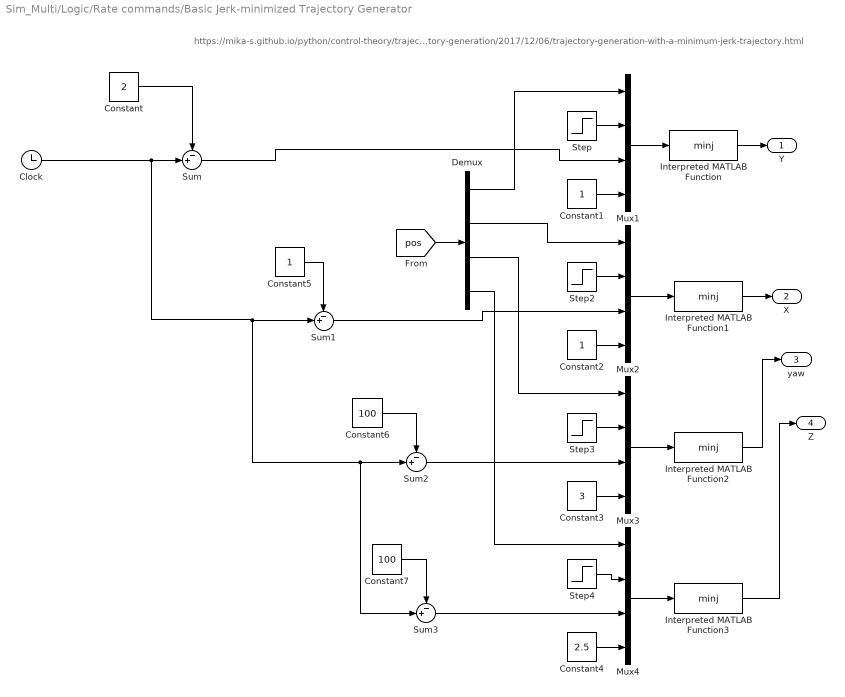
== system Sim_Multi/Logic/Rate commands/Basic Jerk-minimized Trajectory Generator ==
  note: https://mika-s.github.io/python/control-theory/trajectory-generation/2017/12/06/trajectory-generation-with-a-minimum-jerk-trajectory.html
  Clock : Clock
      settings: Decimation=1000
  Constant : Constant  Value=2
  Constant1 : Constant
  Constant2 : Constant
  Constant3 : Constant  Value=3
  Constant4 : Constant  Value=2.5
  Constant5 : Constant
  Constant6 : Constant  Value=100
  Constant7 : Constant  Value=100
  Demux : Demux
  Interpreted MATLAB Function{,1..3} (4 alike) : MATLABFcn  MATLABFcn=minj
  Mux{1..4} (4 alike) : Mux
  Step : Step  Time=2  After=3  SampleTime=0
  Step2 : Step  After=3  SampleTime=0
  Step3 : Step  After=0  SampleTime=0
  Step4 : Step  Before=-1  After=-1  SampleTime=0
  Sum{,1..3} (4 alike) : Sum  Inputs=-+|
  Y : Outport
  X : Outport  Port=2
  yaw : Outport  Port=3
  Z : Outport  Port=4
  wires:
  Interpreted MATLAB Function3/1 -> Z/1
  Constant6/1 -> Sum2/1
  Demux/4 -> Mux4/1
  Demux/3 -> Mux3/1
  Sum1/1 -> Mux2/3
  Clock/1 -> Sum1/2, Sum3/2, Sum2/2, Sum/2
  Constant5/1 -> Sum1/1
  Step4/1 -> Mux4/2
  Sum2/1 -> Mux3/3
  Demux/1 -> Mux1/1
  Sum/1 -> Mux1/3
  Constant1/1 -> Mux1/4
  Constant7/1 -> Sum3/1
  Constant/1 -> Sum/1
  Sum3/1 -> Mux4/3
  Step/1 -> Mux1/2
  Step3/1 -> Mux3/2
  Constant3/1 -> Mux3/4
  Constant4/1 -> Mux4/4
  Mux1/1 -> Interpreted MATLAB Function/1
  [pos] -> Demux/1
  Step2/1 -> Mux2/2
  Mux4/1 -> Interpreted MATLAB Function3/1
  Constant2/1 -> Mux2/4
  Demux/2 -> Mux2/1
  Mux3/1 -> Interpreted MATLAB Function2/1
  Mux2/1 -> Interpreted MATLAB Function1/1
  Interpreted MATLAB Function/1 -> Y/1
  Interpreted MATLAB Function2/1 -> yaw/1
  Interpreted MATLAB Function1/1 -> X/1

== system Sim_Multi/Plant/6DOF model/Body to Inertial ==
  V_b : Inport
  DCM_ib : Inport  Port=2
  Math Function2 : Math  Operator=transpose  SaturateOnIntegerOverflow=on
  Product : Product  Multiplication=Matrix(*)
  Reshape : Reshape  OutputDimensionality=Column vector (2-D)
  Reshape1 : Reshape  OutputDimensionality=Column vector (2-D)
  V_i : Outport
  wires:
  Reshape/1 -> Product/2
  Product/1 -> Reshape1/1
  DCM_ib/1 -> Math Function2/1
  Reshape1/1 -> V_i/1
  V_b/1 -> Reshape/1
  Math Function2/1 -> Product/1  "DCM_bi"

== system Sim_Multi/Plant/6DOF model/Body to Inertial1 ==
  a_b : Inport
  DCM_ib : Inport  Port=2
  Math Function2 : Math  Operator=transpose  SaturateOnIntegerOverflow=on
  Product : Product  Multiplication=Matrix(*)
  Reshape : Reshape  OutputDimensionality=Column vector (2-D)
  Reshape1 : Reshape  OutputDimensionality=Column vector (2-D)
  a_i : Outport
  wires:
  Reshape/1 -> Product/2
  Product/1 -> Reshape1/1
  DCM_ib/1 -> Math Function2/1
  Reshape1/1 -> a_i/1
  a_b/1 -> Reshape/1
  Math Function2/1 -> Product/1  "DCM_bi"

== system Sim_Multi/Plant/6DOF model/Calculate omega_dot ==
  omega [rad/s] : Inport
  Inertia [kgm^2] : Inport  Port=2
  Moments [Nm] : Inport  Port=3
  Cross Product omega x (J * omega) : Subsystem
  Product : Product  Inputs=/*  Multiplication=Matrix(*)
  Reshape : Reshape  OutputDimensionality=Column vector (2-D)
  "Reshape " : Reshape  OutputDimensionality=Column vector (2-D)
  Subsystem : Subsystem
  Sum1 : Sum  Inputs=-+|
  omega_dot [rad/s^2] : Outport
  wires:
  Inertia [kgm^2]/1 -> Product/1, Subsystem/2(J)
  omega [rad/s]/1 -> Cross Product omega x (J * omega)/1(omega), Subsystem/1(omega)
  Subsystem/1(J * omega) -> Cross Product omega x (J * omega)/2(J * omega)
  Cross Product omega x (J * omega)/1(omega x (J * omega)) -> Reshape/1
  Product/1 -> "Reshape "/1
  "Reshape "/1 -> omega_dot [rad/s^2]/1
  Moments [Nm]/1 -> Sum1/2
  Reshape/1 -> Sum1/1
  Sum1/1 -> Product/2

== system Sim_Multi/Plant/6DOF model/Quat Strapdown Eq. ==
  Body_rates : Inport
  Att_init : Inport  Port=2
  -1/2 : Gain  Gain=-0.5
  1/2 : Gain  Gain=0.5
  Cross Product : Subsystem
  Demux : Demux  Outputs=[1 3]
  Dot product : Subsystem
  Mux : Mux  Inputs=[1 3]
  Normalize : Subsystem
  Product : Product  RndMeth=Zero
  Q-Integrator : Integrator  InitialConditionSource=external  InitialCondition=[1 0 0 0]
  Subtract : Sum  Inputs=+-
  rpy2quat : MATLABFcn  MATLABFcn=rpy2quat(u)  OutputDimensions=4
  Att quaternion : Outport
  wires:
  Dot product/1(u.v) -> -1/2/1
  -1/2/1 -> Mux/1
  Body_rates/1 -> Dot product/1(u), Cross Product/1(u), Product/2
  Q-Integrator/1 -> Normalize/1(Input)
  [q123] -> Dot product/2(v)
  Product/1 -> Subtract/1
  Cross Product/1(u x v) -> Subtract/2
  [q0] -> Product/1
  [q123] -> Cross Product/2(v)
  Subtract/1 -> 1/2/1
  1/2/1 -> Mux/2
  Demux/1 -> [q0]
  Demux/2 -> [q123]
  Normalize/1(Output) -> Demux/1, Att quaternion/1
  Mux/1 -> Q-Integrator/1
  rpy2quat/1 -> Q-Integrator/2
  Att_init/1 -> rpy2quat/1

== system Sim_Multi/Plant/6DOF model/Quat to Euler ==
  Quaternion q : Inport
  Fcn : Fcn  Expr=2*(u(3)*u(4)+u(1)*u(2))
  Fcn1 : Fcn  Expr=2*(u(2)*u(4)-u(1)*u(3))
  Fcn2 : Fcn  Expr=2*(u(2)*u(3)+u(1)*u(4))
  Fcn3 : Fcn  Expr=u(1)*u(1)-u(2)*u(2)-u(3)*u(3)+u(4)*u(4)
  Fcn4 : Fcn  Expr=u(1)*u(1)+u(2)*u(2)-u(3)*u(3)-u(4)*u(4)
  Gain : Gain  Gain=-1
  Reshape : Reshape  OutputDimensionality=Column vector (2-D)
  Trigonometric Function : Trigonometry  Operator=asin
  Trigonometric Function1 : Trigonometry  Operator=atan2
  Trigonometric Function2 : Trigonometry  Operator=atan2
  Vector Concatenate : Concatenate  NumInputs=3
  Euler [rad] : Outport
  wires:
  Fcn1/1 -> Trigonometric Function/1
  Trigonometric Function/1 -> Gain/1
  Fcn/1 -> Trigonometric Function1/1
  Fcn3/1 -> Trigonometric Function1/2
  Fcn2/1 -> Trigonometric Function2/1
  Fcn4/1 -> Trigonometric Function2/2
  Trigonometric Function1/1 -> Vector Concatenate/1
  Gain/1 -> Vector Concatenate/2
  Trigonometric Function2/1 -> Vector Concatenate/3
  Quaternion q/1 -> Fcn4/1, Fcn2/1, Fcn/1, Fcn3/1, Fcn1/1
  Vector Concatenate/1 -> Reshape/1
  Reshape/1 -> Euler [rad]/1

== system Sim_Multi/Plant/6DOF model/Quat to Rotation Matrix ==
  Quaternion q : Inport
  Subsystem : Subsystem
  Subsystem1 : Subsystem
  Subsystem2 : Subsystem
  Subsystem3 : Subsystem
  Subsystem4 : Subsystem
  Subsystem5 : Subsystem
  Subsystem6 : Subsystem
  Subsystem7 : Subsystem
  Subsystem8 : Subsystem
  Subsystem9 : Subsystem
  DCM_ib : Outport
  wires:
  Quaternion q/1 -> Subsystem2/1(q), Subsystem8/1(q), Subsystem7/1(q), Subsystem6/1(q), Subsystem1/1(q), Subsystem5/1(q), Subsystem4/1(q), Subsystem3/1(q), Subsystem/1(q)
  Subsystem/1(C_11) -> Subsystem9/1(C_11)
  Subsystem3/1(C_12) -> Subsystem9/2(C_12)
  Subsystem4/1(C_13) -> Subsystem9/3(C_13)
  Subsystem5/1(C_21) -> Subsystem9/4(C_21)
  Subsystem1/1(C_22) -> Subsystem9/5(C_22)
  Subsystem2/1(C_33) -> Subsystem9/9(C_33)
  Subsystem8/1(C_32) -> Subsystem9/8(C_32)
  Subsystem7/1(C_31) -> Subsystem9/7(C_31)
  Subsystem6/1(C_23) -> Subsystem9/6(C_23)
  Subsystem9/1(DCM_ib) -> DCM_ib/1

== system Sim_Multi/Plant/6DOF model/omega x V_b ==
  V_b : Inport
  omega : Inport  Port=2
  Subsystem : Subsystem
  Subsystem1 : Subsystem
  Sum : Sum  Inputs=+|-
  omega x V_b : Outport
  wires:
  Sum/1 -> omega x V_b/1
  omega/1 -> Subsystem1/1(u), Subsystem/1(u)
  V_b/1 -> Subsystem/2(v), Subsystem1/2(v)
  Subsystem/1(Positive elements) -> Sum/1
  Subsystem1/1(Negative elements) -> Sum/2

== system Sim_Multi/Plant/Force//Moment computation/Compute aerodynamic drag of the airframe in Body axes ==
  note: Aerodynamic drag force acting on the airframe
      | The assumption is that the surface area of the airframe from different directions
      | can be described by an ellipsoid. Then the 'acting 'surface area is in the direction
      | of the airspeed vector and can be computed by scaling the airspeed vector so that
      | it points onto the surface of the ellipsoid.
  6DOF dynamics : Inport
  Dynamic parameters : Inport  Port=2
  Aerodynamic drag force : Subsystem
  Bus Selector2 : BusSelector  OutputSignals=V_b,DCM_ib
  Bus Selector3 : BusSelector  OutputSignals=Wind_i,Surface_params
  Total airspeed (Body axes) : Subsystem
  Drag force : Outport
  wires:
  Aerodynamic drag force/1(Drag force (Body axes)) -> Drag force/1
  6DOF dynamics/1 -> Bus Selector2/1
  Dynamic parameters/1 -> Bus Selector3/1
  Bus Selector3/2 -> Aerodynamic drag force/2(Surface_params)  "<Surface_params>"
  Bus Selector2/1 -> Total airspeed (Body axes)/1(V_b)  "<V_b>"
  Bus Selector2/2 -> Total airspeed (Body axes)/2(DCM_ib)  "<DCM_ib>"
  Bus Selector3/1 -> Total airspeed (Body axes)/3(Wind_i)  "<Wind_i>"
  Total airspeed (Body axes)/1(Airspeed (Body)) -> Aerodynamic drag force/1(Airspeed (Body axes))

== system Sim_Multi/Plant/Force//Moment computation/Compute force of gravity in Body axes ==
  note: Force of gravity acting on the airframe
  6DOF dynamics : Inport
  Dynamic parameters : Inport  Port=2
  Bus Selector : BusSelector  OutputSignals=DCM_ib
  Bus Selector1 : BusSelector  OutputSignals=mass_real
  Gravity (Inertial axes) : Constant  Value=[0;0;g]
  Product : Product  Multiplication=Matrix(*)  SaturateOnIntegerOverflow=on  InputSameDT=on  OutDataTypeStr=Inherit: Same as first input
  Product1 : Product
  Reshape : Reshape  OutputDimensionality=Column vector (2-D)
  Gravity force : Outport
  wires:
  Gravity (Inertial axes)/1 -> Product1/1
  Product1/1 -> Product/2  "Force of gravity (Inertial axes)"
  Product/1 -> Reshape/1  "Force of gravity (Body axes)"
  Reshape/1 -> Gravity force/1
  6DOF dynamics/1 -> Bus Selector/1
  Dynamic parameters/1 -> Bus Selector1/1
  Bus Selector1/1 -> Product1/2  "<mass_real>"
  Bus Selector/1 -> Product/1  "<DCM_ib>"

== system Sim_Multi/Plant/Force//Moment computation/Forces and moments generated by spinning propellers ==
  note: Computation of forces and moments for each actuator specified in the initialization routine
  RPM_commands : Inport
  Dynamic parameters : Inport  Port=2
  6DOF dynamics : Inport  Port=3
  Bus Selector : BusSelector  OutputSignals=omega,V_b,DCM_ib
  Bus Selector1 : BusSelector  OutputSignals=Wind_i,MotorMatrix_real,CoG_real
  For Each Subsystem : Subsystem  TreatAsAtomicUnit=on
  Reshape : Reshape  OutputDimensionality=Column vector (2-D)
  Sum of Elements : Sum  Inputs=+  CollapseMode=Specified dimension  CollapseDim=2
  Sum of Elements1 : Sum  Inputs=+  CollapseMode=Specified dimension  CollapseDim=2
  Total airspeed (Body axes) : Subsystem
  Motor moments : Outport
  Motor forces : Outport  Port=2
  tag scope: RPM_motor=global
  wires:
  For Each Subsystem/1(Motor_force) -> Sum of Elements/1
  For Each Subsystem/2(Motor_moment) -> Sum of Elements1/1
  Sum of Elements/1 -> Motor forces/1
  Sum of Elements1/1 -> Motor moments/1
  RPM_commands/1 -> For Each Subsystem/1(RPM_commands)
  6DOF dynamics/1 -> For Each Subsystem/6(6 DOF), Bus Selector/1
  Bus Selector/1 -> For Each Subsystem/2(Body_rates)  "<omega>"
  Dynamic parameters/1 -> Bus Selector1/1
  Bus Selector1/2 -> For Each Subsystem/4(MotorMatrix_real)  "<MotorMatrix_real>"
  Bus Selector1/3 -> For Each Subsystem/5(CoG_real)  "<CoG_real>"
  Bus Selector/2 -> Total airspeed (Body axes)/1(V_b)  "<V_b>"
  Bus Selector/3 -> Total airspeed (Body axes)/2(DCM_ib)  "<DCM_ib>"
  Bus Selector1/1 -> Total airspeed (Body axes)/3(Wind_i)  "<Wind_i>"
  Total airspeed (Body axes)/1(Airspeed (Body)) -> For Each Subsystem/3(Airspeed (Body))
  For Each Subsystem/3(RPM_motor) -> Reshape/1
  Reshape/1 -> [RPM_motor]

== system Sim_Multi/Plant/Force//Moment computation/Ground contact forces and moments in Body axes ==
  note: step 5: output forces and moments (as applied to CoG)
  note: step 4: calculate induced body moment from landing gear
  note: step 3: determine friction force magnitude based on coulmb friction curve
  note: step 2: if below ground, apply penalty method to generate force magnitude
  note: step 1: locate landing gear in inertial frame
  note: position, orientation, velocity (inertial frame), locations of landing gear (body frame), CoG location (body frame)
  note: what we need:
  6DOF dynamics : Inport
  Dynamic parameters : Inport  Port=2
  Ground moments : Outport
  Ground forces : Outport  Port=2
  wires:
  6DOF dynamics/1 -> Ground moments/1
  Dynamic parameters/1 -> Ground forces/1

== system Sim_Multi/State Estimation, Sensors, Noise/Sensor models/Acc noise ==
  Band-Limited White Noise : simulink/Sources/Band-Limited White Noise  Cov=t_sim*57.3*57.3/10000  Ts=t_sim  seed=[25341]
  Constant : Constant  Value=Noise_flag
  Constant1 : Constant  Value=0
  Gain1 : Gain  Gain=0.1
  Gain2 : Gain  Gain=0.08
  Integrator : Integrator
  Rate Transition : RateTransition  OutPortSampleTime=t_sim
  Sum1 : Sum  Inputs=++|
  Switch : Switch  Criteria=u2 > Threshold
  Uniform Random Number : UniformRandomNumber  Minimum=-.001  Maximum=.001  Seed=657  SampleTime=t_sim
  Noise : Outport
  wires:
  Band-Limited White Noise/1 -> Gain2/1
  Uniform Random Number/1 -> Integrator/1
  Integrator/1 -> Gain1/1
  Switch/1 -> Rate Transition/1
  Constant/1 -> Switch/2
  Constant1/1 -> Switch/3
  Gain2/1 -> Sum1/1
  Gain1/1 -> Sum1/2
  Sum1/1 -> Switch/1
  Rate Transition/1 -> Noise/1

== system Sim_Multi/State Estimation, Sensors, Noise/Sensor models/Gyro noise ==
  Band-Limited White Noise : simulink/Sources/Band-Limited White Noise  Cov=t_sim*57.3*57.3/10000  Ts=t_sim  seed=[23341]
  Constant : Constant  Value=Noise_flag
  Constant1 : Constant  Value=0
  Gain1 : Gain  Gain=0.1
  Gain2 : Gain  Gain=0.07
  Integrator : Integrator
  Rate Transition : RateTransition  OutPortSampleTime=t_sim
  Sum1 : Sum  Inputs=++|
  Switch : Switch  Criteria=u2 > Threshold
  Uniform Random Number : UniformRandomNumber  Minimum=-.001  Maximum=.001  Seed=338  SampleTime=t_sim
  Noise : Outport
  wires:
  Band-Limited White Noise/1 -> Gain2/1
  Uniform Random Number/1 -> Integrator/1
  Integrator/1 -> Gain1/1
  Switch/1 -> Rate Transition/1
  Constant/1 -> Switch/2
  Constant1/1 -> Switch/3
  Gain2/1 -> Sum1/1
  Gain1/1 -> Sum1/2
  Sum1/1 -> Switch/1
  Rate Transition/1 -> Noise/1

== system Sim_Multi/State Estimation, Sensors, Noise/State estimation/Normalize ==
  Input : Inport
  Divide : Product  Inputs=*/
  norm : Subsystem
  Output : Outport
  wires:
  Input/1 -> Divide/1, norm/1(u)
  norm/1(||u||) -> Divide/2
  Divide/1 -> Output/1

== system Sim_Multi/State Estimation, Sensors, Noise/State estimation/Normalize1 ==
  Input : Inport
  Divide : Product  Inputs=*/
  norm : Subsystem
  Output : Outport
  wires:
  Input/1 -> Divide/1, norm/1(u)
  norm/1(||u||) -> Divide/2
  Divide/1 -> Output/1

== system Sim_Multi/State Estimation, Sensors, Noise/State estimation/Quat noise ==
  Band-Limited White Noise : simulink/Sources/Band-Limited White Noise  Cov=t_sim*57.3*57.3/10000  Ts=t_sim*30  seed=[23099]
  Constant : Constant  Value=Noise_flag
  Constant1 : Constant  Value=0
  Gain2 : Gain  Gain=0.1
  Rate Transition1 : RateTransition  OutPortSampleTime=t_sim
  Switch : Switch  Criteria=u2 > Threshold
  Noise : Outport
  wires:
  Band-Limited White Noise/1 -> Gain2/1
  Switch/1 -> Noise/1
  Constant/1 -> Switch/2
  Constant1/1 -> Switch/3
  Gain2/1 -> Rate Transition1/1
  Rate Transition1/1 -> Switch/1
